simulink model "mcb_open_loop_control_host_model111"  (R2023b)
settings: Solver=FixedStepDiscrete  StartTime=0.0  StopTime=inf  RelTol=1e-3  EnableMultiTasking=on
InitFcn:
  | if( strcmp(get_param([gcs '/Serial Communication/HW_Selected'], 'Value'), '0'))
  |       set_param([gcs '/Host Serial Setup'], 'BaudRate', '5.625e6');
  | elseif( strcmp(get_param([gcs '/Serial Communication/HW_Selected'], 'Value'), '1'))
  |       set_param([gcs '/Host Serial Setup'], 'BaudRate', '5e6');
  | else
  | 
  | end
values from neighbouring files (symbols this model uses):
  Ts = T_pwm    [mcb_open_loop_control_data.m]
libraries: instrumentseriallib x3
PreSaveFcn:
  | if( strcmp(get_param([gcs '/Serial Communication/HW_Selected'], 'Value'), '0'))
  |       set_param([gcs '/Host Serial Setup'], 'BaudRate', '5.625e6');
  | elseif( strcmp(get_param([gcs '/Serial Communication/HW_Selected'], 'Value'), '1'))
  |       set_param([gcs '/Host Serial Setup'], 'BaudRate', '5e6');
  | else
  | 
  | end
settings Model: Creator=The MathWorks, Inc.  LastModifiedBy=kapis
settings SolverCC: AlgebraicLoopSolver=TrustRegion  MaxZcPerStep=1
settings DataIOCC: LimitDataPoints=on  SaveFormat=Array  ReturnWorkspaceOutputs=off
settings OptimizationCC: LifeSpan=1  EfficientTunableParamExpr=on
settings DebuggingCC: UnderspecifiedInitializationDetection=Classic  MergeDetectMultiDrivingBlocksExec=none  SolverPrmCheckMsg=warning  ParameterPrecisionLossMsg=none  UnconnectedInputMsg=warning  UnconnectedOutputMsg=warning  UnconnectedLineMsg=warning  AllowSymbolicDim=off  PregeneratedLibrarySubsystemCodeDiagnostic=none  SFUnexpectedBacktrackingDiag=warning  SFNoUnconditionalDefaultTransitionDiag=warning  SFExecutionAtInitializationDiag=none  ArithmeticOperatorsInVariantConditions=warning
settings HardwareCC: ProdBitPerPointer=32  ProdLargestAtomicFloat=None  ProdIntDivRoundTo=Undefined  ProdEndianess=Unspecified  ProdWordSize=32  ProdHWDeviceType=32-bit Generic
settings ModelReferenceCC: EnableRefExpFcnMdlSchedulingChecks=on  PropagateSignalLabelsOutOfModel=off
settings SFSimCC: SimUseLocalCustomCode=off  MATLABDynamicMemAlloc=off
settings RTWCC: Description=Real-Time Workshop Embedded Coder  SystemTargetFile=ert.tlc  TemplateMakefile=ert_default_tmf  GenerateReport=on  RTWUseLocalCustomCode=off  IncludeHyperlinkInReport=on  LaunchReport=on  GenerateTraceInfo=on  GenerateTraceReport=on  GenerateTraceReportSl=on  GenerateTraceReportSf=on  GenerateTraceReportEml=on  DLArmComputeVersion=19.05
settings CodeAppCC: IgnoreCustomStorageClasses=off  StateflowObjectComments=on  InternalIdentifier=Classic
settings ERTTargetCC: MultiwordLength=2048  GenerateSampleERTMain=on  ERTCustomFileTemplate=example_file_process.tlc  ConvertIfToSwitch=off  SuppressUnreachableDefaultCases=off
settings ConfigComp: CovMetricSettings=dw  CovSaveCumulativeToWorkspaceVar=on  CovSaveSingleToWorkspaceVar=on  CovExternalEMLEnable=off  CovSFcnEnable=off

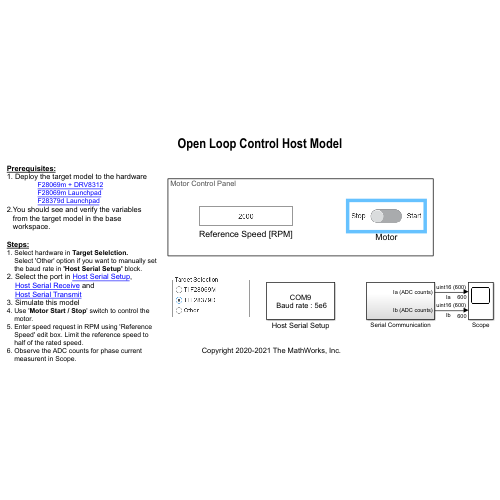
[thumbnail: Simulink's stored preview of the top-level diagram]
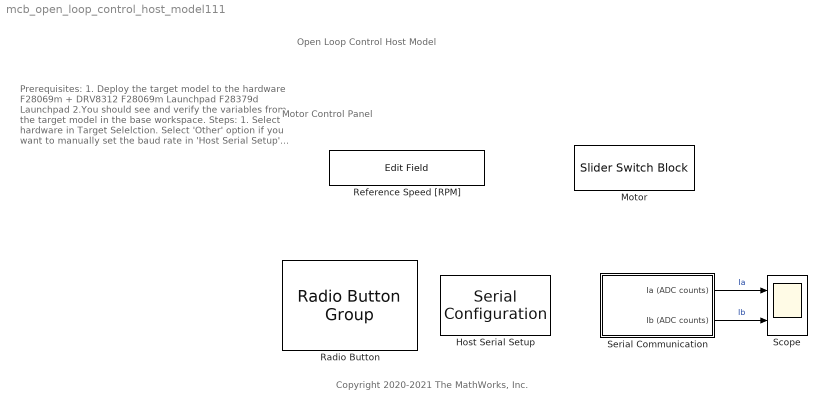
== system mcb_open_loop_control_host_model111 ==
  note: Prerequisites:
      | 1. Deploy the target model to the hardware
      | F28069m + DRV8312
      | F28069m Launchpad
      | F28379d Launchpad
      | 2.You should see and verify the variables
      | from the target model in the base
      | workspace.
      |
      | Steps:
      | 1. Select hardware in Target Selelction.
      | Select 'Other' option if you want to manually set
      | the baud rate in 'Host Serial Setup' block.
      | 2. Select the port in Host Serial Setup ,
      | Host Serial Receive and
      | Host Serial Transmit
      | 3. Simulate this model
      | 4. Use ' Motor Start / Stop ' switch to control the
      | motor.
      | 5. Enter speed request in RPM using 'Reference
      | Speed' edit box. Limit the reference speed to
      | half of the rated speed.
      | 6. Observe the ADC counts for phase current
      | measurent in Scope.
  note: Open Loop Control Host Model
  note: Copyright 2020-2021 The MathWorks, Inc.
  note: Motor Control Panel
  Host Serial Setup : instrumentseriallib/Serial Configuration  Priority=-99  PortSel=COM9  Port=COM9  ComPort=COM9  BaudRate=5e6  DataBits=8  Parity=none  StopBits=1  ByteOrder=little-endian  FlowControl=none  Timeout=2  SimulateUsing=Interpreted execution  BlockInModel=on  aMode=5
  Motor : SliderSwitchBlock  LabelPosition=Hide
      settings: Values={{'Stop', 'Start'}, [0 1]}
  Radio Button : RadioButtonGroup  LabelPosition=Hide  SelectedLabel=TI F28379D  ButtonGroupName=Target Selection
      settings: Values={{'TI F28069M', 'TI F28379D', 'Other'}, [0 1 2]}
  Reference Speed [RPM] : EditField  LabelPosition=Hide  ShowInitialText=on  Alignment=Center
  Scope : Scope  NumInputPorts=2
  Serial Communication : Subsystem
  wires:
  Serial Communication/1(Ia (ADC counts)) -> Scope/1  "Ia"
  Serial Communication/2(Ib (ADC counts)) -> Scope/2  "Ib"

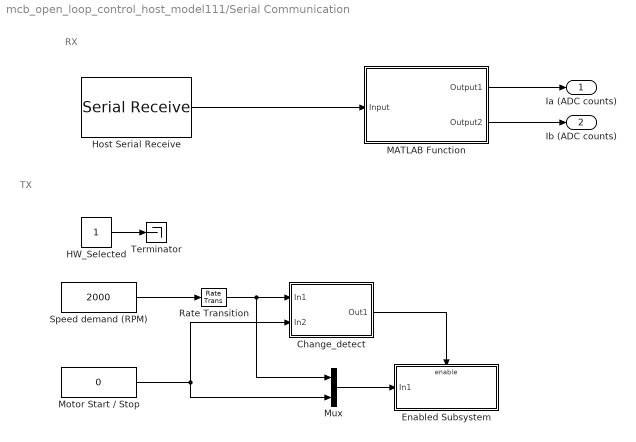
== system mcb_open_loop_control_host_model111/Serial Communication ==
  note: TX
  note: RX
  Change_detect : Subsystem
  Enabled Subsystem : Subsystem  TreatAsAtomicUnit=on
  HW_Selected : Constant  OutDataTypeStr=uint8
  Host Serial Receive : instrumentseriallib/Serial Receive  PortSel=COM9  Port=COM9  ComPort=COM9  DataType=uint16  SaveDataType=uint8  ToggleHeader=on  Header='SS'  ToggleTerminator=on  Terminator=Custom terminator  CustomTerminator='EE'  InputFormat=Row major  ToggleDataSize=on  DataSize=[600 2]  EnableBlockingMode=on  ActionDataUnavailable=Output last received value  ActionWhenDataUnavailable=Output last received value  CustomValue=0  SampleTime=600 * Ts  SimulateUsing=Interpreted execution  BlockInModel=on  aMode=5
  MATLAB Function : MATLAB Function  TreatAsAtomicUnit=on
  Motor Start / Stop : Constant  Value=0  VectorParams1D=off  OutDataTypeStr=single  SampleTime=0.03
  Mux : Mux  Inputs=2
  Rate Transition : RateTransition  OutPortSampleTime=0.03
  Speed demand (RPM) : Constant  Value=2000  VectorParams1D=off  OutDataTypeStr=single  SampleTime=0.03
  Terminator : Terminator
  Ia (ADC counts) : Outport
  Ib (ADC counts) : Outport  Port=2
  wires:
  MATLAB Function/2(Output2) -> Ib (ADC counts)/1
  MATLAB Function/1(Output1) -> Ia (ADC counts)/1
  Host Serial Receive/1 -> MATLAB Function/1(Input)
  HW_Selected/1 -> Terminator/1
  Change_detect/1(Out1) -> Enabled Subsystem/Enable
  Rate Transition/1 -> Mux/1, Change_detect/1(In1)
  Mux/1 -> Enabled Subsystem/1(In1)
  Speed demand (RPM)/1 -> Rate Transition/1
  Motor Start / Stop/1 -> Mux/2, Change_detect/2(In2)

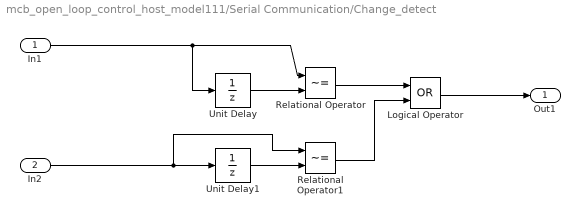
== system mcb_open_loop_control_host_model111/Serial Communication/Change_detect ==
  In1 : Inport
  In2 : Inport  Port=2
  Logical Operator : Logic  Operator=OR  AllPortsSameDT=off  OutDataTypeStr=boolean
  Relational Operator : RelationalOperator  Operator=~=  OutDataTypeStr=boolean  InputSameDT=off
  Relational Operator1 : RelationalOperator  Operator=~=  OutDataTypeStr=boolean  InputSameDT=off
  Unit Delay : UnitDelay  InitialCondition=0.5  SampleTime=-1  HasFrameUpgradeWarning=on
  Unit Delay1 : UnitDelay  SampleTime=-1  HasFrameUpgradeWarning=on
  Out1 : Outport  VectorParamsAs1DForOutWhenUnconnected=off
  wires:
  In2/1 -> Relational Operator1/1, Unit Delay1/1
  Relational Operator1/1 -> Logical Operator/2
  Unit Delay1/1 -> Relational Operator1/2
  Unit Delay/1 -> Relational Operator/2
  In1/1 -> Unit Delay/1, Relational Operator/1
  Relational Operator/1 -> Logical Operator/1
  Logical Operator/1 -> Out1/1

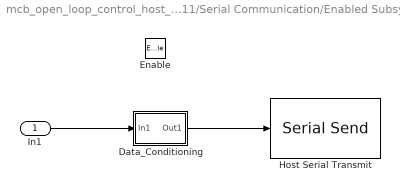
== system mcb_open_loop_control_host_model111/Serial Communication/Enabled Subsystem ==
  In1 : Inport
  Enable : EnablePort
  Data_Conditioning : Subsystem
  Host Serial Transmit : instrumentseriallib/Serial Send  PortSel=COM9  Port=COM9  ComPort=COM9  Header=[]  Terminator=<none>  CustomTerminator=[]  EnableBlockingMode=off  SimulateUsing=Interpreted execution  BlockInModel=on  aMode=5
  wires:
  In1/1 -> Data_Conditioning/1(In1)
  Data_Conditioning/1(Out1) -> Host Serial Transmit/1

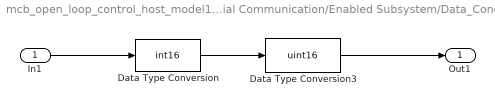
== system mcb_open_loop_control_host_model111/Serial Communication/Enabled Subsystem/Data_Conditioning ==
  In1 : Inport
  Data Type Conversion : DataTypeConversion  OutDataTypeStr=int16  RndMeth=Simplest  SaturateOnIntegerOverflow=off
  Data Type Conversion3 : DataTypeConversion  OutDataTypeStr=uint16  ConvertRealWorld=Stored Integer (SI)  RndMeth=Simplest  SaturateOnIntegerOverflow=off
  Out1 : Outport  VectorParamsAs1DForOutWhenUnconnected=off
  wires:
  In1/1 -> Data Type Conversion/1
  Data Type Conversion3/1 -> Out1/1
  Data Type Conversion/1 -> Data Type Conversion3/1

== matlab function mcb_open_loop_control_host_model111/Serial Communication/MATLAB Function ==
  data: Output1 output; Output2 output; Input input
function [ Output1, Output2] = unBuf(Input)

Output1= Input(:, 1);
Output2 = Input(:, 2);
end
